simulink model "ALL_SET_GET_SETUP_Funcitons_Library_2020a"  (R2021b)
settings: Solver=VariableStepAuto  StartTime=0.0  StopTime=inf  RelTol=1e-3
(part 2 of 3)

== system ALL_SET_GET_SETUP_Funcitons_Library_2020a/Get_Functions/GetOutputPwmFrequencyKhz ==
  Address : Inport
  S-Function Builder56 : S-Function  Priority=3  FunctionName=GetOutputPwmFrequencyKhz  SFunctionModules=GetOutputPwmFrequencyKhz_wrapper  SFunctionDeploymentMode=off  EnableBusSupport=off  mask(S-Function Builder){}
      mask help: Simulink:masks:SFunctionBuilder_MD
      mask init: same as ALL_SET_GET_SETUP_Funcitons_Library_2020a/Get_Functions/Get3PhaseMotorAngle/S-Function Builder87
      settings: CopyFcn=set_param(gcbh,'LinkStatus','none')  OpenFcn=sfunctionwizard(gcbh)
      mask Display: plot(val(:,1),val(:,2)),disp(sys),port_label('input',1,'Address'),port_label('output',1,'Result'),port_label('output',2,'Error')
  Result : Outport
  Error : Outport  Port=2
  wires:
  S-Function Builder56/1 -> Result/1
  Address/1 -> S-Function Builder56/1
  S-Function Builder56/2 -> Error/1

== system ALL_SET_GET_SETUP_Funcitons_Library_2020a/Get_Functions/GetPhaseACurrent ==
  Address : Inport
  S-Function Builder49 : S-Function  Priority=3  FunctionName=GetPhaseACurrent  SFunctionModules=GetPhaseACurrent_wrapper  SFunctionDeploymentMode=off  EnableBusSupport=off  mask(S-Function Builder){}
      mask help: Simulink:masks:SFunctionBuilder_MD
      mask init: same as ALL_SET_GET_SETUP_Funcitons_Library_2020a/Get_Functions/Get3PhaseMotorAngle/S-Function Builder87
      settings: CopyFcn=set_param(gcbh,'LinkStatus','none')  OpenFcn=sfunctionwizard(gcbh)
      mask Display:
      | plot(val(:,1),val(:,2))
      | disp(sys)
      | port_label('input',1,'Address')
      | port_label('output',1,'Result')
      | port_label('output',2,'Error')
  Result : Outport
  Error : Outport  Port=2
  wires:
  S-Function Builder49/2 -> Error/1
  S-Function Builder49/1 -> Result/1
  Address/1 -> S-Function Builder49/1

== system ALL_SET_GET_SETUP_Funcitons_Library_2020a/Get_Functions/GetPhaseAVoltage ==
  Address : Inport
  S-Function Builder47 : S-Function  Priority=3  FunctionName=GetPhaseAVoltage  SFunctionModules=GetPhaseAVoltage_wrapper  SFunctionDeploymentMode=off  EnableBusSupport=off  mask(S-Function Builder){}
      mask help: Simulink:masks:SFunctionBuilder_MD
      mask init: same as ALL_SET_GET_SETUP_Funcitons_Library_2020a/Get_Functions/Get3PhaseMotorAngle/S-Function Builder87
      settings: CopyFcn=set_param(gcbh,'LinkStatus','none')  OpenFcn=sfunctionwizard(gcbh)
      mask Display: plot(val(:,1),val(:,2)),disp(sys),port_label('input',1,'Address'),port_label('output',1,'Result'),port_label('output',2,'Error')
  Result : Outport
  Error : Outport  Port=2
  wires:
  S-Function Builder47/1 -> Result/1
  Address/1 -> S-Function Builder47/1
  S-Function Builder47/2 -> Error/1

== system ALL_SET_GET_SETUP_Funcitons_Library_2020a/Get_Functions/GetPhaseBCurrent ==
  Address : Inport
  S-Function Builder50 : S-Function  Priority=3  FunctionName=GetPhaseBCurrent  SFunctionModules=GetPhaseBCurrent_wrapper  SFunctionDeploymentMode=off  EnableBusSupport=off  mask(S-Function Builder){}
      mask help: Simulink:masks:SFunctionBuilder_MD
      mask init: same as ALL_SET_GET_SETUP_Funcitons_Library_2020a/Get_Functions/Get3PhaseMotorAngle/S-Function Builder87
      settings: CopyFcn=set_param(gcbh,'LinkStatus','none')  OpenFcn=sfunctionwizard(gcbh)
      mask Display:
      | plot(val(:,1),val(:,2))
      | disp(sys)
      | port_label('input',1,'Address')
      | port_label('output',1,'Result')
      | port_label('output',2,'Error')
  Result : Outport
  Error : Outport  Port=2
  wires:
  S-Function Builder50/2 -> Error/1
  Address/1 -> S-Function Builder50/1
  S-Function Builder50/1 -> Result/1

== system ALL_SET_GET_SETUP_Funcitons_Library_2020a/Get_Functions/GetPhaseBVoltage ==
  Address : Inport
  S-Function Builder48 : S-Function  Priority=3  FunctionName=GetPhaseBVoltage  SFunctionModules=GetPhaseBVoltage_wrapper  SFunctionDeploymentMode=off  EnableBusSupport=off  mask(S-Function Builder){}
      mask help: Simulink:masks:SFunctionBuilder_MD
      mask init: same as ALL_SET_GET_SETUP_Funcitons_Library_2020a/Get_Functions/Get3PhaseMotorAngle/S-Function Builder87
      settings: CopyFcn=set_param(gcbh,'LinkStatus','none')  OpenFcn=sfunctionwizard(gcbh)
      mask Display:
      | plot(val(:,1),val(:,2))
      | disp(sys)
      | port_label('input',1,'Address')
      | port_label('output',1,'Result')
      | port_label('output',2,'Error')
  Result : Outport
  Error : Outport  Port=2
  wires:
  S-Function Builder48/2 -> Error/1
  S-Function Builder48/1 -> Result/1
  Address/1 -> S-Function Builder48/1

== system ALL_SET_GET_SETUP_Funcitons_Library_2020a/Get_Functions/GetPositionControllerKi ==
  Address : Inport
  S-Function Builder72 : S-Function  Priority=3  FunctionName=GetPositionControllerKi  SFunctionModules=GetPositionControllerKi_wrapper  SFunctionDeploymentMode=off  EnableBusSupport=off  mask(S-Function Builder){}
      mask help: Simulink:masks:SFunctionBuilder_MD
      mask init: same as ALL_SET_GET_SETUP_Funcitons_Library_2020a/Get_Functions/Get3PhaseMotorAngle/S-Function Builder87
      settings: CopyFcn=set_param(gcbh,'LinkStatus','none')  OpenFcn=sfunctionwizard(gcbh)
      mask Display:
      | plot(val(:,1),val(:,2))
      | disp(sys)
      | port_label('input',1,'Address')
      | port_label('output',1,'Result')
      | port_label('output',2,'Error')
  Result : Outport
  Error : Outport  Port=2
  wires:
  Address/1 -> S-Function Builder72/1
  S-Function Builder72/2 -> Error/1
  S-Function Builder72/1 -> Result/1

== system ALL_SET_GET_SETUP_Funcitons_Library_2020a/Get_Functions/GetPositionControllerKp ==
  Address : Inport
  S-Function Builder71 : S-Function  Priority=3  FunctionName=GetPositionControllerKp  SFunctionModules=GetPositionControllerKp_wrapper  SFunctionDeploymentMode=off  EnableBusSupport=off  mask(S-Function Builder){}
      mask help: Simulink:masks:SFunctionBuilder_MD
      mask init: same as ALL_SET_GET_SETUP_Funcitons_Library_2020a/Get_Functions/Get3PhaseMotorAngle/S-Function Builder87
      settings: CopyFcn=set_param(gcbh,'LinkStatus','none')  OpenFcn=sfunctionwizard(gcbh)
      mask Display: plot(val(:,1),val(:,2)),disp(sys),port_label('input',1,'Address'),port_label('output',1,'Result'),port_label('output',2,'Error')
  Result : Outport
  Error : Outport  Port=2
  wires:
  S-Function Builder71/2 -> Error/1
  S-Function Builder71/1 -> Result/1
  Address/1 -> S-Function Builder71/1

== system ALL_SET_GET_SETUP_Funcitons_Library_2020a/Get_Functions/GetPositionCountsFeedback ==
  Address : Inport
  S-Function Builder73 : S-Function  Priority=3  FunctionName=GetPositionCountsFeedback  SFunctionModules=GetPositionCountsFeedback_wrapper  SFunctionDeploymentMode=off  EnableBusSupport=off  mask(S-Function Builder){}
      mask help: Simulink:masks:SFunctionBuilder_MD
      mask init: same as ALL_SET_GET_SETUP_Funcitons_Library_2020a/Get_Functions/Get3PhaseMotorAngle/S-Function Builder87
      settings: CopyFcn=set_param(gcbh,'LinkStatus','none')  OpenFcn=sfunctionwizard(gcbh)
      mask Display: plot(val(:,1),val(:,2)),disp(sys),port_label('input',1,'Address'),port_label('output',1,'Result'),port_label('output',2,'Error')
  Result : Outport
  Error : Outport  Port=2
  wires:
  Address/1 -> S-Function Builder73/1
  S-Function Builder73/2 -> Error/1
  S-Function Builder73/1 -> Result/1

== system ALL_SET_GET_SETUP_Funcitons_Library_2020a/Get_Functions/GetPositionRef ==
  Address : Inport
  S-Function Builder80 : S-Function  Priority=3  FunctionName=GetPositionReference  SFunctionModules=GetPositionReference_wrapper  SFunctionDeploymentMode=off  EnableBusSupport=off  mask(S-Function Builder){}
      mask help: Simulink:masks:SFunctionBuilder_MD
      mask init: same as ALL_SET_GET_SETUP_Funcitons_Library_2020a/Get_Functions/Get3PhaseMotorAngle/S-Function Builder87
      settings: CopyFcn=set_param(gcbh,'LinkStatus','none')  OpenFcn=sfunctionwizard(gcbh)
      mask Display:
      | plot(val(:,1),val(:,2))
      | disp(sys)
      | port_label('input',1,'Address')
      | port_label('output',1,'Result')
      | port_label('output',2,'Error')
  Result : Outport
  Error : Outport  Port=2
  wires:
  S-Function Builder80/1 -> Result/1
  Address/1 -> S-Function Builder80/1
  S-Function Builder80/2 -> Error/1

== system ALL_SET_GET_SETUP_Funcitons_Library_2020a/Get_Functions/GetPowerRef ==
  Address : Inport
  S-Function Builder79 : S-Function  Priority=3  FunctionName=GetPowerReference  SFunctionModules=GetPowerReference_wrapper  SFunctionDeploymentMode=off  EnableBusSupport=off  mask(S-Function Builder){}
      mask help: Simulink:masks:SFunctionBuilder_MD
      mask init: same as ALL_SET_GET_SETUP_Funcitons_Library_2020a/Get_Functions/Get3PhaseMotorAngle/S-Function Builder87
      settings: CopyFcn=set_param(gcbh,'LinkStatus','none')  OpenFcn=sfunctionwizard(gcbh)
      mask Display:
      | plot(val(:,1),val(:,2))
      | disp(sys)
      | port_label('input',1,'Address')
      | port_label('output',1,'Result')
      | port_label('output',2,'Error')
  Result : Outport
  Error : Outport  Port=2
  wires:
  Address/1 -> S-Function Builder79/1
  S-Function Builder79/1 -> Result/1
  S-Function Builder79/2 -> Error/1

== system ALL_SET_GET_SETUP_Funcitons_Library_2020a/Get_Functions/GetQuadratureCurrentIqFeedback ==
  Address : Inport
  S-Function Builder57 : S-Function  Priority=3  FunctionName=GetQuadratureCurrentIqFeedback  SFunctionModules=GetQuadratureCurrentIqFeedback_wrapper  SFunctionDeploymentMode=off  EnableBusSupport=off  mask(S-Function Builder){}
      mask help: Simulink:masks:SFunctionBuilder_MD
      mask init: same as ALL_SET_GET_SETUP_Funcitons_Library_2020a/Get_Functions/Get3PhaseMotorAngle/S-Function Builder87
      settings: CopyFcn=set_param(gcbh,'LinkStatus','none')  OpenFcn=sfunctionwizard(gcbh)
      mask Display: plot(val(:,1),val(:,2)),disp(sys),port_label('input',1,'Address'),port_label('output',1,'Result'),port_label('output',2,'Error')
  Result : Outport
  Error : Outport  Port=2
  wires:
  S-Function Builder57/2 -> Error/1
  Address/1 -> S-Function Builder57/1
  S-Function Builder57/1 -> Result/1

== system ALL_SET_GET_SETUP_Funcitons_Library_2020a/Get_Functions/GetSpeedAccelerationValue ==
  Address : Inport
  S-Function Builder91 : S-Function  Priority=3  FunctionName=GetSpeedAccelerationValue  SFunctionModules=GetSpeedAccelerationValue_wrapper  SFunctionDeploymentMode=off  EnableBusSupport=off  mask(S-Function Builder){}
      mask help: Simulink:masks:SFunctionBuilder_MD
      mask init: same as ALL_SET_GET_SETUP_Funcitons_Library_2020a/Get_Functions/Get3PhaseMotorAngle/S-Function Builder87
      settings: CopyFcn=set_param(gcbh,'LinkStatus','none')  OpenFcn=sfunctionwizard(gcbh)
      mask Display:
      | plot(val(:,1),val(:,2))
      | disp(sys)
      | port_label('input',1,'Address')
      | port_label('output',1,'Result')
      | port_label('output',2,'Error')
  Result : Outport
  Error : Outport  Port=2
  wires:
  S-Function Builder91/1 -> Result/1
  Address/1 -> S-Function Builder91/1
  S-Function Builder91/2 -> Error/1

== system ALL_SET_GET_SETUP_Funcitons_Library_2020a/Get_Functions/GetSpeedControllerKi ==
  Address : Inport
  S-Function Builder55 : S-Function  Priority=3  FunctionName=GetSpeedControllerKi  SFunctionModules=GetSpeedControllerKi_wrapper  SFunctionDeploymentMode=off  EnableBusSupport=off  mask(S-Function Builder){}
      mask help: Simulink:masks:SFunctionBuilder_MD
      mask init: same as ALL_SET_GET_SETUP_Funcitons_Library_2020a/Get_Functions/Get3PhaseMotorAngle/S-Function Builder87
      settings: CopyFcn=set_param(gcbh,'LinkStatus','none')  OpenFcn=sfunctionwizard(gcbh)
      mask Display:
      | plot(val(:,1),val(:,2))
      | disp(sys)
      | port_label('input',1,'Address')
      | port_label('output',1,'Result')
      | port_label('output',2,'Error')
  Result : Outport
  Error : Outport  Port=2
  wires:
  S-Function Builder55/2 -> Error/1
  Address/1 -> S-Function Builder55/1
  S-Function Builder55/1 -> Result/1

== system ALL_SET_GET_SETUP_Funcitons_Library_2020a/Get_Functions/GetSpeedControllerKp ==
  Address : Inport
  S-Function Builder54 : S-Function  Priority=3  FunctionName=GetSpeedControllerKp  SFunctionModules=GetSpeedControllerKp_wrapper  SFunctionDeploymentMode=off  EnableBusSupport=off  mask(S-Function Builder){}
      mask help: Simulink:masks:SFunctionBuilder_MD
      mask init: same as ALL_SET_GET_SETUP_Funcitons_Library_2020a/Get_Functions/Get3PhaseMotorAngle/S-Function Builder87
      settings: CopyFcn=set_param(gcbh,'LinkStatus','none')  OpenFcn=sfunctionwizard(gcbh)
      mask Display:
      | plot(val(:,1),val(:,2))
      | disp(sys)
      | port_label('input',1,'Address')
      | port_label('output',1,'Result')
      | port_label('output',2,'Error')
  Result : Outport
  Error : Outport  Port=2
  wires:
  S-Function Builder54/2 -> Error/1
  Address/1 -> S-Function Builder54/1
  S-Function Builder54/1 -> Result/1

== system ALL_SET_GET_SETUP_Funcitons_Library_2020a/Get_Functions/GetSpeedDecelerationValue ==
  Address : Inport
  S-Function Builder92 : S-Function  Priority=3  FunctionName=GetSpeedDecelerationValue  SFunctionModules=GetSpeedDecelerationValue_wrapper  SFunctionDeploymentMode=off  EnableBusSupport=off  mask(S-Function Builder){}
      mask help: Simulink:masks:SFunctionBuilder_MD
      mask init: same as ALL_SET_GET_SETUP_Funcitons_Library_2020a/Get_Functions/Get3PhaseMotorAngle/S-Function Builder87
      settings: CopyFcn=set_param(gcbh,'LinkStatus','none')  OpenFcn=sfunctionwizard(gcbh)
      mask Display:
      | plot(val(:,1),val(:,2))
      | disp(sys)
      | port_label('input',1,'Address')
      | port_label('output',1,'Result')
      | port_label('output',2,'Error')
  Result : Outport
  Error : Outport  Port=2
  wires:
  S-Function Builder92/1 -> Result/1
  Address/1 -> S-Function Builder92/1
  S-Function Builder92/2 -> Error/1

== system ALL_SET_GET_SETUP_Funcitons_Library_2020a/Get_Functions/GetSpeedFeedback ==
  Address : Inport
  S-Function Builder66 : S-Function  Priority=3  FunctionName=GetSpeedFeedback  SFunctionModules=GetSpeedFeedback_wrapper  SFunctionDeploymentMode=off  EnableBusSupport=off  mask(S-Function Builder){}
      mask help: Simulink:masks:SFunctionBuilder_MD
      mask init: same as ALL_SET_GET_SETUP_Funcitons_Library_2020a/Get_Functions/Get3PhaseMotorAngle/S-Function Builder87
      settings: CopyFcn=set_param(gcbh,'LinkStatus','none')  OpenFcn=sfunctionwizard(gcbh)
      mask Display: plot(val(:,1),val(:,2)),disp(sys),port_label('input',1,'Address'),port_label('output',1,'Result'),port_label('output',2,'Error')
  Result : Outport
  Error : Outport  Port=2
  wires:
  Address/1 -> S-Function Builder66/1
  S-Function Builder66/1 -> Result/1
  S-Function Builder66/2 -> Error/1

== system ALL_SET_GET_SETUP_Funcitons_Library_2020a/Get_Functions/GetSpeedLimit ==
  Address : Inport
  S-Function Builder70 : S-Function  Priority=3  FunctionName=GetSpeedLimit  SFunctionModules=GetSpeedLimit_wrapper  SFunctionDeploymentMode=off  EnableBusSupport=off  mask(S-Function Builder){}
      mask help: Simulink:masks:SFunctionBuilder_MD
      mask init: same as ALL_SET_GET_SETUP_Funcitons_Library_2020a/Get_Functions/Get3PhaseMotorAngle/S-Function Builder87
      settings: CopyFcn=set_param(gcbh,'LinkStatus','none')  OpenFcn=sfunctionwizard(gcbh)
      mask Display:
      | plot(val(:,1),val(:,2))
      | disp(sys)
      | port_label('input',1,'Address')
      | port_label('output',1,'Result')
      | port_label('output',2,'Error')
  Result : Outport
  Out2 : Outport  Port=2
  wires:
  Address/1 -> S-Function Builder70/1
  S-Function Builder70/2 -> Out2/1
  S-Function Builder70/1 -> Result/1

== system ALL_SET_GET_SETUP_Funcitons_Library_2020a/Get_Functions/GetSpeedRef ==
  Address : Inport
  S-Function Builder78 : S-Function  Priority=3  FunctionName=GetSpeedReference  SFunctionModules=GetSpeedReference_wrapper  SFunctionDeploymentMode=off  EnableBusSupport=off  mask(S-Function Builder){}
      mask help: Simulink:masks:SFunctionBuilder_MD
      mask init: same as ALL_SET_GET_SETUP_Funcitons_Library_2020a/Get_Functions/Get3PhaseMotorAngle/S-Function Builder87
      settings: CopyFcn=set_param(gcbh,'LinkStatus','none')  OpenFcn=sfunctionwizard(gcbh)
      mask Display:
      | plot(val(:,1),val(:,2))
      | disp(sys)
      | port_label('input',1,'Address')
      | port_label('output',1,'Result')
      | port_label('output',2,'Error')
  Result : Outport
  Error : Outport  Port=2
  wires:
  S-Function Builder78/2 -> Error/1
  S-Function Builder78/1 -> Result/1
  Address/1 -> S-Function Builder78/1

== system ALL_SET_GET_SETUP_Funcitons_Library_2020a/Get_Functions/GetTorqueRefIq ==
  Address : Inport
  S-Function Builder7 : S-Function  Priority=3  FunctionName=GetTorqueReferenceIq  SFunctionModules=GetTorqueReferenceIq_wrapper  SFunctionDeploymentMode=off  EnableBusSupport=off  mask(S-Function Builder){}
      mask help: Simulink:masks:SFunctionBuilder_MD
      mask init: same as ALL_SET_GET_SETUP_Funcitons_Library_2020a/Get_Functions/Get3PhaseMotorAngle/S-Function Builder87
      settings: CopyFcn=set_param(gcbh,'LinkStatus','none')  OpenFcn=sfunctionwizard(gcbh)
      mask Display: plot(val(:,1),val(:,2)),disp(sys),port_label('input',1,'Address'),port_label('output',1,'Result'),port_label('output',2,'Error')
  Result : Outport
  Error : Outport  Port=2
  wires:
  S-Function Builder7/2 -> Error/1
  Address/1 -> S-Function Builder7/1
  S-Function Builder7/1 -> Result/1

== system ALL_SET_GET_SETUP_Funcitons_Library_2020a/Get_Functions/GetUartBaudrate ==
  Address : Inport
  S-Function Builder90 : S-Function  Priority=3  FunctionName=GetUartBaudrate  SFunctionModules=GetUartBaudrate_wrapper  SFunctionDeploymentMode=off  EnableBusSupport=off  mask(S-Function Builder){}
      mask help: Simulink:masks:SFunctionBuilder_MD
      mask init: same as ALL_SET_GET_SETUP_Funcitons_Library_2020a/Get_Functions/Get3PhaseMotorAngle/S-Function Builder87
      settings: CopyFcn=set_param(gcbh,'LinkStatus','none')  OpenFcn=sfunctionwizard(gcbh)
      mask Display:
      | plot(val(:,1),val(:,2))
      | disp(sys)
      | port_label('input',1,'Address')
      | port_label('output',1,'Result')
      | port_label('output',2,'Error')
  Result : Outport
  Error : Outport  Port=2
  wires:
  S-Function Builder90/2 -> Error/1
  Address/1 -> S-Function Builder90/1
  S-Function Builder90/1 -> Result/1

== system ALL_SET_GET_SETUP_Funcitons_Library_2020a/SET_Fucntions/EmergencyStop ==
  note: Error
  Address : Inport
  Display22 : Display
      settings: Format=decimal (Stored Integer)
  Display23 : Display
      settings: Format=decimal (Stored Integer)
  S-Function Builder11 : S-Function  Priority=2  FunctionName=EmergencyStop  SFunctionModules=EmergencyStop_wrapper  SFunctionDeploymentMode=off  EnableBusSupport=off  mask(S-Function Builder){}
      mask help: Simulink:masks:SFunctionBuilder_MD
      mask init: same as ALL_SET_GET_SETUP_Funcitons_Library_2020a/Get_Functions/Get3PhaseMotorAngle/S-Function Builder87
      settings: CopyFcn=set_param(gcbh,'LinkStatus','none')  OpenFcn=sfunctionwizard(gcbh)
      mask Display:
      | plot(val(:,1),val(:,2))
      | disp(sys)
      | port_label('input',1,'Address')
      | port_label('output',1,'Result')
      | port_label('output',2,'Error')
  Result : Outport
  Error : Outport  Port=2
  wires:
  S-Function Builder11/2 -> Error/1, Display23/1
  S-Function Builder11/1 -> Result/1, Display22/1
  Address/1 -> S-Function Builder11/1

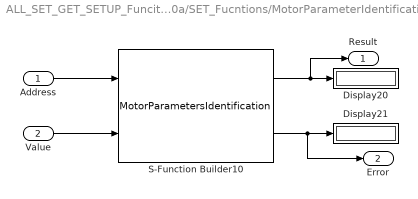
== system ALL_SET_GET_SETUP_Funcitons_Library_2020a/SET_Fucntions/MotorParameterIdentification ==
  Address : Inport
  Value : Inport  Port=2
  Display20 : Display
      settings: Format=decimal (Stored Integer)
  Display21 : Display
      settings: Format=decimal (Stored Integer)
  S-Function Builder10 : S-Function  Priority=2  FunctionName=MotorParametersIdentification  SFunctionModules=MotorParametersIdentification_wrapper  SFunctionDeploymentMode=off  EnableBusSupport=off  mask(S-Function Builder){}
      mask help: Simulink:masks:SFunctionBuilder_MD
      mask init: same as ALL_SET_GET_SETUP_Funcitons_Library_2020a/Get_Functions/Get3PhaseMotorAngle/S-Function Builder87
      settings: CopyFcn=set_param(gcbh,'LinkStatus','none')  OpenFcn=sfunctionwizard(gcbh)
      mask Display:
      | plot(val(:,1),val(:,2))
      | disp(sys)
      | port_label('input',1,'Address')
      | port_label('input',2,'Value')
      | port_label('output',1,'Result')
      | port_label('output',2,'Error')
  Result : Outport
  Error : Outport  Port=2
  wires:
  S-Function Builder10/2 -> Error/1, Display21/1
  S-Function Builder10/1 -> Result/1, Display20/1
  Value/1 -> S-Function Builder10/2
  Address/1 -> S-Function Builder10/1

== system ALL_SET_GET_SETUP_Funcitons_Library_2020a/SET_Fucntions/OverwriteErrorRegister ==
  Address : Inport
  Display68 : Display
      settings: Format=decimal (Stored Integer)
  Display69 : Display
      settings: Format=decimal (Stored Integer)
  S-Function Builder34 : S-Function  Priority=2  FunctionName=OverwriteErrorRegister  SFunctionModules=OverwriteErrorRegister_wrapper  SFunctionDeploymentMode=off  EnableBusSupport=off  mask(S-Function Builder){}
      mask help: Simulink:masks:SFunctionBuilder_MD
      mask init: same as ALL_SET_GET_SETUP_Funcitons_Library_2020a/Get_Functions/Get3PhaseMotorAngle/S-Function Builder87
      settings: CopyFcn=set_param(gcbh,'LinkStatus','none')  OpenFcn=sfunctionwizard(gcbh)
      mask Display:
      | plot(val(:,1),val(:,2))
      | disp(sys)
      | port_label('input',1,'Address')
      | port_label('output',1,'Result')
      | port_label('output',2,'Error')
  Result : Outport
  Error : Outport  Port=2
  wires:
  S-Function Builder34/1 -> Result/1, Display68/1
  S-Function Builder34/2 -> Error/1, Display69/1
  Address/1 -> S-Function Builder34/1

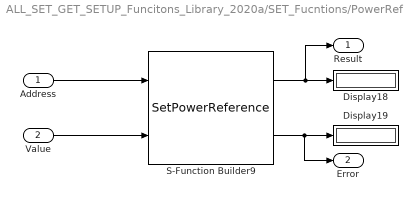
== system ALL_SET_GET_SETUP_Funcitons_Library_2020a/SET_Fucntions/PowerRef ==
  Address : Inport
  Value : Inport  Port=2
  Display18 : Display
      settings: Format=decimal (Stored Integer)
  Display19 : Display
      settings: Format=decimal (Stored Integer)
  S-Function Builder9 : S-Function  Priority=2  FunctionName=SetPowerReference  SFunctionModules=SetPowerReference_wrapper  SFunctionDeploymentMode=off  EnableBusSupport=off  mask(S-Function Builder){}
      mask help: Simulink:masks:SFunctionBuilder_MD
      mask init: same as ALL_SET_GET_SETUP_Funcitons_Library_2020a/Get_Functions/Get3PhaseMotorAngle/S-Function Builder87
      settings: CopyFcn=set_param(gcbh,'LinkStatus','none')  OpenFcn=sfunctionwizard(gcbh)
      mask Display:
      | plot(val(:,1),val(:,2))
      | disp(sys)
      | port_label('input',1,'Address')
      | port_label('input',2,'Value')
      | port_label('output',1,'Result')
      | port_label('output',2,'Error')
  Result : Outport
  Error : Outport  Port=2
  wires:
  S-Function Builder9/1 -> Result/1, Display18/1
  S-Function Builder9/2 -> Error/1, Display19/1
  Address/1 -> S-Function Builder9/1
  Value/1 -> S-Function Builder9/2

== system ALL_SET_GET_SETUP_Funcitons_Library_2020a/SET_Fucntions/ResetDevice Address ==
  Address : Inport
  Display44 : Display
      settings: Format=decimal (Stored Integer)
  Display45 : Display
      settings: Format=decimal (Stored Integer)
  S-Function Builder22 : S-Function  Priority=2  FunctionName=ResetDeviceAddress  SFunctionModules=ResetDeviceAddress_wrapper  SFunctionDeploymentMode=off  EnableBusSupport=off  mask(S-Function Builder){}
      mask help: Simulink:masks:SFunctionBuilder_MD
      mask init: same as ALL_SET_GET_SETUP_Funcitons_Library_2020a/Get_Functions/Get3PhaseMotorAngle/S-Function Builder87
      settings: CopyFcn=set_param(gcbh,'LinkStatus','none')  OpenFcn=sfunctionwizard(gcbh)
      mask Display:
      | plot(val(:,1),val(:,2))
      | disp(sys)
      | port_label('input',1,'Address')
      | port_label('output',1,'Result')
      | port_label('output',2,'Error')
  Result : Outport
  Error : Outport  Port=2
  wires:
  Address/1 -> S-Function Builder22/1
  S-Function Builder22/2 -> Display45/1, Error/1
  S-Function Builder22/1 -> Result/1, Display44/1

== system ALL_SET_GET_SETUP_Funcitons_Library_2020a/SET_Fucntions/ResetFactory ==
  Address : Inport
  Display48 : Display
      settings: Format=decimal (Stored Integer)
  Display49 : Display
      settings: Format=decimal (Stored Integer)
  S-Function Builder24 : S-Function  Priority=2  FunctionName=ResetFactory  SFunctionModules=ResetFactory_wrapper  SFunctionDeploymentMode=off  EnableBusSupport=off  mask(S-Function Builder){}
      mask help: Simulink:masks:SFunctionBuilder_MD
      mask init: same as ALL_SET_GET_SETUP_Funcitons_Library_2020a/Get_Functions/Get3PhaseMotorAngle/S-Function Builder87
      settings: CopyFcn=set_param(gcbh,'LinkStatus','none')  OpenFcn=sfunctionwizard(gcbh)
      mask Display:
      | plot(val(:,1),val(:,2))
      | disp(sys)
      | port_label('input',1,'Address')
      | port_label('output',1,'Result')
      | port_label('output',2,'Error')
  Result : Outport
  Error : Outport  Port=2
  wires:
  S-Function Builder24/2 -> Error/1, Display49/1
  S-Function Builder24/1 -> Result/1, Display48/1
  Address/1 -> S-Function Builder24/1

== system ALL_SET_GET_SETUP_Funcitons_Library_2020a/SET_Fucntions/ResetPositiontoZero ==
  Address : Inport
  Display66 : Display
      settings: Format=decimal (Stored Integer)
  Display67 : Display
      settings: Format=decimal (Stored Integer)
  S-Function Builder33 : S-Function  Priority=2  FunctionName=ResetPositionToZero  SFunctionModules=ResetPositionToZero_wrapper  SFunctionDeploymentMode=off  EnableBusSupport=off  mask(S-Function Builder){}
      mask help: Simulink:masks:SFunctionBuilder_MD
      mask init: same as ALL_SET_GET_SETUP_Funcitons_Library_2020a/Get_Functions/Get3PhaseMotorAngle/S-Function Builder87
      settings: CopyFcn=set_param(gcbh,'LinkStatus','none')  OpenFcn=sfunctionwizard(gcbh)
      mask Display:
      | plot(val(:,1),val(:,2))
      | disp(sys)
      | port_label('input',1,'Address')
      | port_label('output',1,'Result')
      | port_label('output',2,'Error')
  Result : Outport
  Error : Outport  Port=2
  wires:
  S-Function Builder33/1 -> Result/1, Display66/1
  S-Function Builder33/2 -> Error/1, Display67/1
  Address/1 -> S-Function Builder33/1

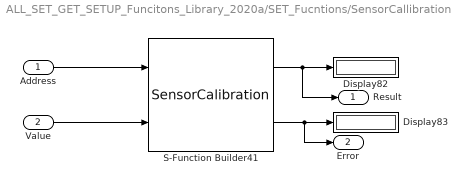
== system ALL_SET_GET_SETUP_Funcitons_Library_2020a/SET_Fucntions/SensorCallibration ==
  Address : Inport
  Value : Inport  Port=2
  Display82 : Display
      settings: Format=decimal (Stored Integer)
  Display83 : Display
      settings: Format=decimal (Stored Integer)
  S-Function Builder41 : S-Function  Priority=2  FunctionName=SensorCalibration  SFunctionModules=SensorCalibration_wrapper  SFunctionDeploymentMode=off  EnableBusSupport=off  mask(S-Function Builder){}
      mask help: Simulink:masks:SFunctionBuilder_MD
      mask init: same as ALL_SET_GET_SETUP_Funcitons_Library_2020a/Get_Functions/Get3PhaseMotorAngle/S-Function Builder87
      settings: CopyFcn=set_param(gcbh,'LinkStatus','none')  OpenFcn=sfunctionwizard(gcbh)
      mask Display:
      | plot(val(:,1),val(:,2))
      | disp(sys)
      | port_label('input',1,'Address')
      | port_label('input',2,'Value')
      | port_label('output',1,'Result')
      | port_label('output',2,'Error')
  Result : Outport
  Error : Outport  Port=2
  wires:
  Value/1 -> S-Function Builder41/2
  S-Function Builder41/1 -> Result/1, Display82/1
  Address/1 -> S-Function Builder41/1
  S-Function Builder41/2 -> Error/1, Display83/1

== system ALL_SET_GET_SETUP_Funcitons_Library_2020a/SET_Fucntions/SetCanBusBaudrate ==
  Address : Inport
  Value : Inport  Port=2
  S-Function Builder46 : S-Function  Priority=2  FunctionName=SetCanbusBoudrate  SFunctionModules=SetCanbusBoudrate_wrapper  SFunctionDeploymentMode=off  EnableBusSupport=off  mask(S-Function Builder){}
      mask help: Simulink:masks:SFunctionBuilder_MD
      mask init: same as ALL_SET_GET_SETUP_Funcitons_Library_2020a/Get_Functions/Get3PhaseMotorAngle/S-Function Builder87
      settings: CopyFcn=set_param(gcbh,'LinkStatus','none')  OpenFcn=sfunctionwizard(gcbh)
      mask Display:
      | plot(val(:,1),val(:,2))
      | disp(sys)
      | port_label('input',1,'Address')
      | port_label('input',2,'Value')
      | port_label('output',1,'Result')
      | port_label('output',2,'Error')
  Result : Outport
  Error : Outport  Port=2
  wires:
  Address/1 -> S-Function Builder46/1
  Value/1 -> S-Function Builder46/2
  S-Function Builder46/2 -> Error/1
  S-Function Builder46/1 -> Result/1

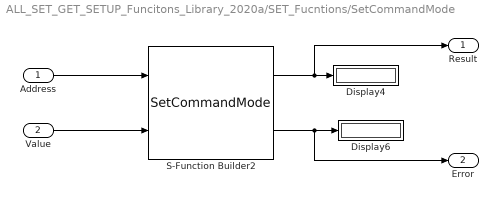
== system ALL_SET_GET_SETUP_Funcitons_Library_2020a/SET_Fucntions/SetCommandMode ==
  Address : Inport  OutDataTypeStr=uint8  LockScale=on
  Value : Inport  Port=2  OutDataTypeStr=boolean  LockScale=on
  Display4 : Display
      settings: Format=decimal (Stored Integer)
  Display6 : Display
      settings: Format=decimal (Stored Integer)
  S-Function Builder2 : S-Function  Priority=2  FunctionName=SetCommandMode  SFunctionModules=SetCommandMode_wrapper  SFunctionDeploymentMode=off  EnableBusSupport=off  mask(S-Function Builder){}
      mask help: Simulink:masks:SFunctionBuilder_MD
      mask init: same as ALL_SET_GET_SETUP_Funcitons_Library_2020a/Get_Functions/Get3PhaseMotorAngle/S-Function Builder87
      settings: CopyFcn=set_param(gcbh,'LinkStatus','none')  OpenFcn=sfunctionwizard(gcbh)
      mask Display: plot(val(:,1),val(:,2)),disp(sys),port_label('input',1,'Address'),port_label('input',2,'Value'),port_label('output',1,'Result'),port_label('output',2,'Error')
  Result : Outport  OutDataTypeStr=boolean
  Error : Outport  Port=2  OutDataTypeStr=boolean
  wires:
  S-Function Builder2/1 -> Result/1, Display4/1
  S-Function Builder2/2 -> Error/1, Display6/1
  Address/1 -> S-Function Builder2/1
  Value/1 -> S-Function Builder2/2

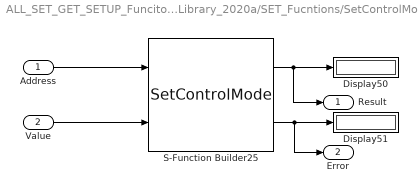
== system ALL_SET_GET_SETUP_Funcitons_Library_2020a/SET_Fucntions/SetControlMode ==
  Address : Inport
  Value : Inport  Port=2
  Display50 : Display
      settings: Format=decimal (Stored Integer)
  Display51 : Display
      settings: Format=decimal (Stored Integer)
  S-Function Builder25 : S-Function  Priority=2  FunctionName=SetControlMode  SFunctionModules=SetControlMode_wrapper  SFunctionDeploymentMode=off  EnableBusSupport=off  mask(S-Function Builder){}
      mask help: Simulink:masks:SFunctionBuilder_MD
      mask init: same as ALL_SET_GET_SETUP_Funcitons_Library_2020a/Get_Functions/Get3PhaseMotorAngle/S-Function Builder87
      settings: CopyFcn=set_param(gcbh,'LinkStatus','none')  OpenFcn=sfunctionwizard(gcbh)
      mask Display: plot(val(:,1),val(:,2)),disp(sys),port_label('input',1,'Address'),port_label('input',2,'Value'),port_label('output',1,'Result'),port_label('output',2,'Error')
  Result : Outport
  Error : Outport  Port=2
  wires:
  S-Function Builder25/1 -> Result/1, Display50/1
  S-Function Builder25/2 -> Error/1, Display51/1
  Value/1 -> S-Function Builder25/2
  Address/1 -> S-Function Builder25/1

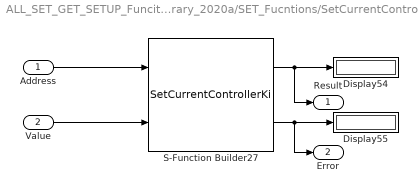
== system ALL_SET_GET_SETUP_Funcitons_Library_2020a/SET_Fucntions/SetCurrentControlKi ==
  Address : Inport
  Value : Inport  Port=2
  Display54 : Display
      settings: Format=decimal (Stored Integer)
  Display55 : Display
      settings: Format=decimal (Stored Integer)
  S-Function Builder27 : S-Function  Priority=2  FunctionName=SetCurrentControllerKi  SFunctionModules=SetCurrentControllerKi_wrapper  SFunctionDeploymentMode=off  EnableBusSupport=off  mask(S-Function Builder){}
      mask help: Simulink:masks:SFunctionBuilder_MD
      mask init: same as ALL_SET_GET_SETUP_Funcitons_Library_2020a/Get_Functions/Get3PhaseMotorAngle/S-Function Builder87
      settings: CopyFcn=set_param(gcbh,'LinkStatus','none')  OpenFcn=sfunctionwizard(gcbh)
      mask Display:
      | plot(val(:,1),val(:,2))
      | disp(sys)
      | port_label('input',1,'Address')
      | port_label('input',2,'Value')
      | port_label('output',1,'Result')
      | port_label('output',2,'Error')
  Result : Outport
  Error : Outport  Port=2
  wires:
  Value/1 -> S-Function Builder27/2
  S-Function Builder27/1 -> Result/1, Display54/1
  S-Function Builder27/2 -> Error/1, Display55/1
  Address/1 -> S-Function Builder27/1

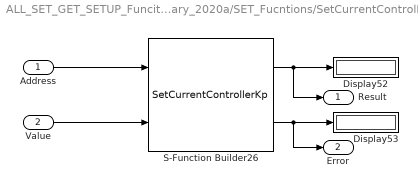
== system ALL_SET_GET_SETUP_Funcitons_Library_2020a/SET_Fucntions/SetCurrentControlKp ==
  Address : Inport
  Value : Inport  Port=2
  Display52 : Display
      settings: Format=decimal (Stored Integer)
  Display53 : Display
      settings: Format=decimal (Stored Integer)
  S-Function Builder26 : S-Function  Priority=2  FunctionName=SetCurrentControllerKp  SFunctionModules=SetCurrentControllerKp_wrapper  SFunctionDeploymentMode=off  EnableBusSupport=off  mask(S-Function Builder){}
      mask help: Simulink:masks:SFunctionBuilder_MD
      mask init: same as ALL_SET_GET_SETUP_Funcitons_Library_2020a/Get_Functions/Get3PhaseMotorAngle/S-Function Builder87
      settings: CopyFcn=set_param(gcbh,'LinkStatus','none')  OpenFcn=sfunctionwizard(gcbh)
      mask Display:
      | plot(val(:,1),val(:,2))
      | disp(sys)
      | port_label('input',1,'Address')
      | port_label('input',2,'Value')
      | port_label('output',1,'Result')
      | port_label('output',2,'Error')
  Result : Outport
  Error : Outport  Port=2
  wires:
  Value/1 -> S-Function Builder26/2
  S-Function Builder26/1 -> Result/1, Display52/1
  Address/1 -> S-Function Builder26/1
  S-Function Builder26/2 -> Error/1, Display53/1

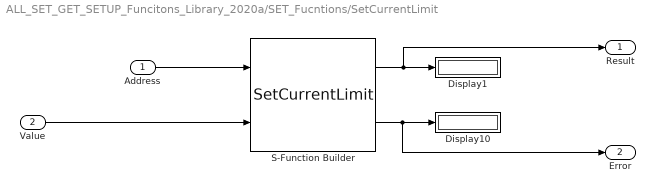
== system ALL_SET_GET_SETUP_Funcitons_Library_2020a/SET_Fucntions/SetCurrentLimit ==
  Address : Inport  Tag=Address  LockScale=on
  Value : Inport  Port=2  LockScale=on
  Display1 : Display
      settings: Format=decimal (Stored Integer)
  Display10 : Display
      settings: Format=decimal (Stored Integer)
  S-Function Builder : S-Function  Priority=2  FunctionName=SetCurrentLimit  SFunctionModules=SetCurrentLimit_wrapper  SFunctionDeploymentMode=off  EnableBusSupport=off  mask(S-Function Builder){}
      mask help: Simulink:masks:SFunctionBuilder_MD
      mask init: same as ALL_SET_GET_SETUP_Funcitons_Library_2020a/Get_Functions/Get3PhaseMotorAngle/S-Function Builder87
      settings: CopyFcn=set_param(gcbh,'LinkStatus','none')  OpenFcn=sfunctionwizard(gcbh)
      mask Display: plot(val(:,1),val(:,2)),disp(sys),port_label('input',1,'Address'),port_label('input',2,'Value'),port_label('output',1,'Result'),port_label('output',2,'Error')
  Result : Outport  OutDataTypeStr=boolean
  Error : Outport  Port=2  OutDataTypeStr=int32
  wires:
  Value/1 -> S-Function Builder/2
  S-Function Builder/2 -> Error/1, Display10/1
  S-Function Builder/1 -> Result/1, Display1/1
  Address/1 -> S-Function Builder/1

== system ALL_SET_GET_SETUP_Funcitons_Library_2020a/SET_Fucntions/SetDeviceAddress ==
  Address : Inport
  Value : Inport  Port=2
  S-Function Builder1 : S-Function  Priority=2  FunctionName=SetDeviceAddress  SFunctionModules=SetDeviceAddress_wrapper  SFunctionDeploymentMode=off  EnableBusSupport=off  mask(S-Function Builder){}
      mask help: Simulink:masks:SFunctionBuilder_MD
      mask init: same as ALL_SET_GET_SETUP_Funcitons_Library_2020a/Get_Functions/Get3PhaseMotorAngle/S-Function Builder87
      settings: CopyFcn=set_param(gcbh,'LinkStatus','none')  OpenFcn=sfunctionwizard(gcbh)
      mask Display:
      | plot(val(:,1),val(:,2))
      | disp(sys)
      | port_label('input',1,'Address')
      | port_label('input',2,'Value')
      | port_label('output',1,'Result')
      | port_label('output',2,'Error')
  Result : Outport
  Error : Outport  Port=2
  wires:
  S-Function Builder1/2 -> Error/1
  Value/1 -> S-Function Builder1/2
  S-Function Builder1/1 -> Result/1
  Address/1 -> S-Function Builder1/1

== system ALL_SET_GET_SETUP_Funcitons_Library_2020a/SET_Fucntions/SetEncoderHallCcwOffset ==
  Address : Inport
  Value : Inport  Port=2
  Display84 : Display
      settings: Format=decimal (Stored Integer)
  Display85 : Display
      settings: Format=decimal (Stored Integer)
  S-Function Builder42 : S-Function  Priority=2  FunctionName=SetEncoderHallCcwOffset  SFunctionModules=SetEncoderHallCcwOffset_wrapper  SFunctionDeploymentMode=off  EnableBusSupport=off  mask(S-Function Builder){}
      mask help: Simulink:masks:SFunctionBuilder_MD
      mask init: same as ALL_SET_GET_SETUP_Funcitons_Library_2020a/Get_Functions/Get3PhaseMotorAngle/S-Function Builder87
      settings: CopyFcn=set_param(gcbh,'LinkStatus','none')  OpenFcn=sfunctionwizard(gcbh)
      mask Display: plot(val(:,1),val(:,2)),disp(sys),port_label('input',1,'Address'),port_label('input',2,'Value'),port_label('output',1,'Result'),port_label('output',2,'Error')
  Result : Outport
  Error : Outport  Port=2
  wires:
  S-Function Builder42/2 -> Error/1, Display85/1
  Value/1 -> S-Function Builder42/2
  S-Function Builder42/1 -> Result/1, Display84/1
  Address/1 -> S-Function Builder42/1

== system ALL_SET_GET_SETUP_Funcitons_Library_2020a/SET_Fucntions/SetEncoderHallCwOffset ==
  Address : Inport
  Value : Inport  Port=2
  S-Function Builder43 : S-Function  Priority=2  FunctionName=SetEncoderHallCwOffset  SFunctionModules=SetEncoderHallCwOffset_wrapper  SFunctionDeploymentMode=off  EnableBusSupport=off  mask(S-Function Builder){}
      mask help: Simulink:masks:SFunctionBuilder_MD
      mask init: same as ALL_SET_GET_SETUP_Funcitons_Library_2020a/Get_Functions/Get3PhaseMotorAngle/S-Function Builder87
      settings: CopyFcn=set_param(gcbh,'LinkStatus','none')  OpenFcn=sfunctionwizard(gcbh)
      mask Display:
      | plot(val(:,1),val(:,2))
      | disp(sys)
      | port_label('input',1,'Address')
      | port_label('input',2,'Value')
      | port_label('output',1,'Result')
      | port_label('output',2,'Error')
  Result : Outport
  Error : Outport  Port=2
  wires:
  Address/1 -> S-Function Builder43/1
  S-Function Builder43/2 -> Error/1
  S-Function Builder43/1 -> Result/1
  Value/1 -> S-Function Builder43/2

== system ALL_SET_GET_SETUP_Funcitons_Library_2020a/SET_Fucntions/SetEncoderLines ==
  Address : Inport
  Value : Inport  Port=2
  Display38 : Display
      settings: Format=decimal (Stored Integer)
  Display39 : Display
      settings: Format=decimal (Stored Integer)
  S-Function Builder19 : S-Function  Priority=2  FunctionName=SetIncrementalEncoderLines  SFunctionModules=SetIncrementalEncoderLines_wrapper  SFunctionDeploymentMode=off  EnableBusSupport=off  mask(S-Function Builder){}
      mask help: Simulink:masks:SFunctionBuilder_MD
      mask init: same as ALL_SET_GET_SETUP_Funcitons_Library_2020a/Get_Functions/Get3PhaseMotorAngle/S-Function Builder87
      settings: CopyFcn=set_param(gcbh,'LinkStatus','none')  OpenFcn=sfunctionwizard(gcbh)
      mask Display:
      | plot(val(:,1),val(:,2))
      | disp(sys)
      | port_label('input',1,'Address')
      | port_label('input',2,'Value')
      | port_label('output',1,'Result')
      | port_label('output',2,'Error')
  Result : Outport
  Error : Outport  Port=2
  wires:
  S-Function Builder19/1 -> Result/1, Display38/1
  Value/1 -> S-Function Builder19/2
  S-Function Builder19/2 -> Error/1, Display39/1
  Address/1 -> S-Function Builder19/1

== system ALL_SET_GET_SETUP_Funcitons_Library_2020a/SET_Fucntions/SetFeedBackControlMode ==
  Address : Inport
  Value : Inport  Port=2
  Display42 : Display
      settings: Format=decimal (Stored Integer)
  Display43 : Display
      settings: Format=decimal (Stored Integer)
  S-Function Builder21 : S-Function  Priority=2  FunctionName=SetFeedbackControlMode  SFunctionModules=SetFeedbackControlMode_wrapper  SFunctionDeploymentMode=off  EnableBusSupport=off  mask(S-Function Builder){}
      mask help: Simulink:masks:SFunctionBuilder_MD
      mask init: same as ALL_SET_GET_SETUP_Funcitons_Library_2020a/Get_Functions/Get3PhaseMotorAngle/S-Function Builder87
      settings: CopyFcn=set_param(gcbh,'LinkStatus','none')  OpenFcn=sfunctionwizard(gcbh)
      mask Display:
      | plot(val(:,1),val(:,2))
      | disp(sys)
      | port_label('input',1,'Address')
      | port_label('input',2,'Value')
      | port_label('output',1,'Result')
      | port_label('output',2,'Error')
  Result : Outport
  Error : Outport  Port=2
  wires:
  S-Function Builder21/1 -> Result/1, Display42/1
  S-Function Builder21/2 -> Error/1, Display43/1
  Value/1 -> S-Function Builder21/2
  Address/1 -> S-Function Builder21/1

== system ALL_SET_GET_SETUP_Funcitons_Library_2020a/SET_Fucntions/SetFilterGainBldcPmsm ==
  Address : Inport
  Value : Inport  Port=2
  Display76 : Display
      settings: Format=decimal (Stored Integer)
  Display77 : Display
      settings: Format=decimal (Stored Integer)
  S-Function Builder38 : S-Function  Priority=2  FunctionName=SetFilterGainBldcPmsm  SFunctionModules=SetFilterGainBldcPmsm_wrapper  SFunctionDeploymentMode=off  EnableBusSupport=off  mask(S-Function Builder){}
      mask help: Simulink:masks:SFunctionBuilder_MD
      mask init: same as ALL_SET_GET_SETUP_Funcitons_Library_2020a/Get_Functions/Get3PhaseMotorAngle/S-Function Builder87
      settings: CopyFcn=set_param(gcbh,'LinkStatus','none')  OpenFcn=sfunctionwizard(gcbh)
      mask Display: plot(val(:,1),val(:,2)),disp(sys),port_label('input',1,'Address'),port_label('input',2,'Value'),port_label('output',1,'Result'),port_label('output',2,'Error')
  Result : Outport
  Error : Outport  Port=2
  wires:
  S-Function Builder38/2 -> Error/1, Display77/1
  S-Function Builder38/1 -> Result/1, Display76/1
  Address/1 -> S-Function Builder38/1
  Value/1 -> S-Function Builder38/2

== system ALL_SET_GET_SETUP_Funcitons_Library_2020a/SET_Fucntions/SetFilterGainBldcPmsmUltrafast ==
  Address : Inport
  Value : Inport  Port=2
  Display78 : Display
      settings: Format=decimal (Stored Integer)
  Display79 : Display
      settings: Format=decimal (Stored Integer)
  S-Function Builder39 : S-Function  Priority=2  FunctionName=SetFilterGainBldcPmsmUltrafast  SFunctionModules=SetFilterGainBldcPmsmUltrafast_wrapper  SFunctionDeploymentMode=off  EnableBusSupport=off  mask(S-Function Builder){}
      mask help: Simulink:masks:SFunctionBuilder_MD
      mask init: same as ALL_SET_GET_SETUP_Funcitons_Library_2020a/Get_Functions/Get3PhaseMotorAngle/S-Function Builder87
      settings: CopyFcn=set_param(gcbh,'LinkStatus','none')  OpenFcn=sfunctionwizard(gcbh)
      mask Display: plot(val(:,1),val(:,2)),disp(sys),port_label('input',1,'Address'),port_label('input',2,'Value'),port_label('output',1,'Result'),port_label('output',2,'Error')
  Result : Outport
  Error : Outport  Port=2
  wires:
  S-Function Builder39/2 -> Error/1, Display79/1
  S-Function Builder39/1 -> Result/1, Display78/1
  Address/1 -> S-Function Builder39/1
  Value/1 -> S-Function Builder39/2

== system ALL_SET_GET_SETUP_Funcitons_Library_2020a/SET_Fucntions/SetMagnetizingCurrentIdReference ==
  Address : Inport
  Value : Inport  Port=2
  Display58 : Display
      settings: Format=decimal (Stored Integer)
  Display59 : Display
      settings: Format=decimal (Stored Integer)
  S-Function Builder29 : S-Function  Priority=2  FunctionName=SetMagnetizingCurrentIdReference  SFunctionModules=SetMagnetizingCurrentIdReference_wrapper  SFunctionDeploymentMode=off  EnableBusSupport=off  mask(S-Function Builder){}
      mask help: Simulink:masks:SFunctionBuilder_MD
      mask init: same as ALL_SET_GET_SETUP_Funcitons_Library_2020a/Get_Functions/Get3PhaseMotorAngle/S-Function Builder87
      settings: CopyFcn=set_param(gcbh,'LinkStatus','none')  OpenFcn=sfunctionwizard(gcbh)
      mask Display: plot(val(:,1),val(:,2)),disp(sys),port_label('input',1,'Address'),port_label('input',2,'Value'),port_label('output',1,'Result'),port_label('output',2,'Error')
  Result : Outport
  Error : Outport  Port=2
  wires:
  S-Function Builder29/1 -> Result/1, Display58/1
  S-Function Builder29/2 -> Error/1, Display59/1
  Address/1 -> S-Function Builder29/1
  Value/1 -> S-Function Builder29/2

== system ALL_SET_GET_SETUP_Funcitons_Library_2020a/SET_Fucntions/SetMonitoringMode ==
  Address : Inport
  Value : Inport  Port=2
  Display56 : Display
      settings: Format=decimal (Stored Integer)
  Display57 : Display
      settings: Format=decimal (Stored Integer)
  S-Function Builder28 : S-Function  Priority=2  FunctionName=SetMonitoringMode  SFunctionModules=SetMonitoringMode_wrapper  SFunctionDeploymentMode=off  EnableBusSupport=off  mask(S-Function Builder){}
      mask help: Simulink:masks:SFunctionBuilder_MD
      mask init: same as ALL_SET_GET_SETUP_Funcitons_Library_2020a/Get_Functions/Get3PhaseMotorAngle/S-Function Builder87
      settings: CopyFcn=set_param(gcbh,'LinkStatus','none')  OpenFcn=sfunctionwizard(gcbh)
      mask Display:
      | plot(val(:,1),val(:,2))
      | disp(sys)
      | port_label('input',1,'Address')
      | port_label('input',2,'Value')
      | port_label('output',1,'Result')
      | port_label('output',2,'Error')
  Result : Outport
  Error : Outport  Port=2
  wires:
  S-Function Builder28/2 -> Error/1, Display57/1
  Address/1 -> S-Function Builder28/1
  S-Function Builder28/1 -> Result/1, Display56/1
  Value/1 -> S-Function Builder28/2

== system ALL_SET_GET_SETUP_Funcitons_Library_2020a/SET_Fucntions/SetMotorDirection ==
  Address : Inport
  Value : Inport  Port=2
  Display30 : Display  Commented=on
      settings: Format=decimal (Stored Integer)
  Display31 : Display  Commented=on
      settings: Format=decimal (Stored Integer)
  S-Function Builder15 : S-Function  Priority=2  Commented=on  FunctionName=SetMotorDirection  SFunctionModules=SetMotorDirection_wrapper  SFunctionDeploymentMode=off  EnableBusSupport=off  mask(S-Function Builder){}
      mask help: Simulink:masks:SFunctionBuilder_MD
      mask init: same as ALL_SET_GET_SETUP_Funcitons_Library_2020a/Get_Functions/Get3PhaseMotorAngle/S-Function Builder87
      settings: CopyFcn=set_param(gcbh,'LinkStatus','none')  OpenFcn=sfunctionwizard(gcbh)
      mask Display: plot(val(:,1),val(:,2)),disp(sys),port_label('input',1,'Address'),port_label('input',2,'Value'),port_label('output',1,'Result'),port_label('output',2,'Error')
  Result : Outport
  Error : Outport  Port=2
  wires:
  S-Function Builder15/2 -> Error/1, Display31/1
  Value/1 -> S-Function Builder15/2
  S-Function Builder15/1 -> Result/1, Display30/1
  Address/1 -> S-Function Builder15/1

== system ALL_SET_GET_SETUP_Funcitons_Library_2020a/SET_Fucntions/SetMotorInductance ==
  Address : Inport
  Value : Inport  Port=2
  Display34 : Display
      settings: Format=decimal (Stored Integer)
  Display35 : Display
      settings: Format=decimal (Stored Integer)
  S-Function Builder17 : S-Function  Priority=2  FunctionName=SetMotorInductance  SFunctionModules=SetMotorInductance_wrapper  SFunctionDeploymentMode=off  EnableBusSupport=off  mask(S-Function Builder){}
      mask help: Simulink:masks:SFunctionBuilder_MD
      mask init: same as ALL_SET_GET_SETUP_Funcitons_Library_2020a/Get_Functions/Get3PhaseMotorAngle/S-Function Builder87
      settings: CopyFcn=set_param(gcbh,'LinkStatus','none')  OpenFcn=sfunctionwizard(gcbh)
      mask Display:
      | plot(val(:,1),val(:,2))
      | disp(sys)
      | port_label('input',1,'Address')
      | port_label('input',2,'Value')
      | port_label('output',1,'Result')
      | port_label('output',2,'Error')
  Result : Outport
  Error : Outport  Port=2
  wires:
  S-Function Builder17/1 -> Result/1, Display34/1
  S-Function Builder17/2 -> Error/1, Display35/1
  Value/1 -> S-Function Builder17/2
  Address/1 -> S-Function Builder17/1

== system ALL_SET_GET_SETUP_Funcitons_Library_2020a/SET_Fucntions/SetMotorPoleCounts ==
  Address : Inport
  Value : Inport  Port=2
  Display36 : Display
      settings: Format=decimal (Stored Integer)
  Display37 : Display
      settings: Format=decimal (Stored Integer)
  S-Function Builder18 : S-Function  Priority=2  FunctionName=SetMotorPolesCounts  SFunctionModules=SetMotorPolesCounts_wrapper  SFunctionDeploymentMode=off  EnableBusSupport=off  mask(S-Function Builder){}
      mask help: Simulink:masks:SFunctionBuilder_MD
      mask init: same as ALL_SET_GET_SETUP_Funcitons_Library_2020a/Get_Functions/Get3PhaseMotorAngle/S-Function Builder87
      settings: CopyFcn=set_param(gcbh,'LinkStatus','none')  OpenFcn=sfunctionwizard(gcbh)
      mask Display:
      | plot(val(:,1),val(:,2))
      | disp(sys)
      | port_label('input',1,'Address')
      | port_label('input',2,'Value')
      | port_label('output',1,'Result')
      | port_label('output',2,'Error')
  Result : Outport
  Error : Outport  Port=2
  wires:
  S-Function Builder18/1 -> Result/1, Display36/1
  Value/1 -> S-Function Builder18/2
  S-Function Builder18/2 -> Error/1, Display37/1
  Address/1 -> S-Function Builder18/1

== system ALL_SET_GET_SETUP_Funcitons_Library_2020a/SET_Fucntions/SetMotorResistance ==
  Address : Inport
  Value : Inport  Port=2
  Display32 : Display
      settings: Format=decimal (Stored Integer)
  Display33 : Display
      settings: Format=decimal (Stored Integer)
  S-Function Builder16 : S-Function  Priority=2  FunctionName=SetMotorResistance  SFunctionModules=SetMotorResistance_wrapper  SFunctionDeploymentMode=off  EnableBusSupport=off  mask(S-Function Builder){}
      mask help: Simulink:masks:SFunctionBuilder_MD
      mask init: same as ALL_SET_GET_SETUP_Funcitons_Library_2020a/Get_Functions/Get3PhaseMotorAngle/S-Function Builder87
      settings: CopyFcn=set_param(gcbh,'LinkStatus','none')  OpenFcn=sfunctionwizard(gcbh)
      mask Display: plot(val(:,1),val(:,2)),disp(sys),port_label('input',1,'Address'),port_label('input',2,'Value'),port_label('output',1,'Result'),port_label('output',2,'Error')
  Result : Outport
  Error : Outport  Port=2
  wires:
  S-Function Builder16/1 -> Result/1, Display32/1
  S-Function Builder16/2 -> Error/1, Display33/1
  Address/1 -> S-Function Builder16/1
  Value/1 -> S-Function Builder16/2
